simulink model "DC_motor_model"  (R2020b)
settings: Solver=ode45  StartTime=0.0  StopTime=5  RelTol=1e-3
values from neighbouring files (symbols this model uses):
  ctrl =     [DATA.mat]
  daq =     [DATA.mat]
  drv =     [DATA.mat]
  gbox =     [DATA.mat]
  mld =     [DATA.mat]
  mot =     [DATA.mat]
  rads2rpm = 9.54929658551    [DATA.mat]
  sens =     [DATA.mat]
undefined symbols (not defined in the file or in its folder): step_size
settings Model: Creator=gioel  LastModifiedBy=gioel
settings DataIOCC: ReturnWorkspaceOutputs=off

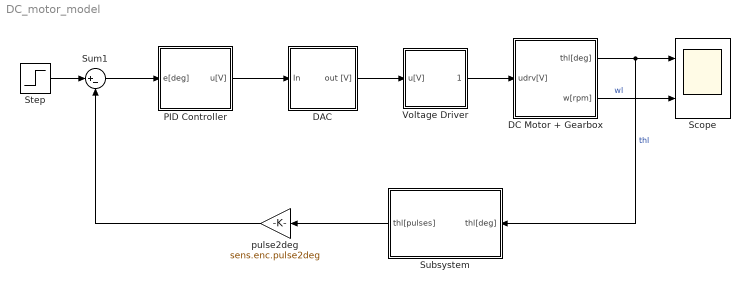
== system DC_motor_model ==
  DAC : Subsystem
  DC Motor + Gearbox : Subsystem
  PID Controller : Subsystem
  Scope : Scope  NumInputPorts=2
  Step : Step  After=step_size  SampleTime=0
  Subsystem : Subsystem
  Sum1 : Sum  Inputs=|+-
  Voltage Driver : Subsystem
  pulse2deg : Gain  Gain=sens.enc.pulse2deg
  wires:
  DAC/1(out [V]) -> Voltage Driver/1(u[V])
  Voltage Driver/1(udrv[V]) -> DC Motor + Gearbox/1(udrv[V])
  DC Motor + Gearbox/1(thl[deg]) -> Subsystem/1(thl[deg]), Scope/1  "thl"
  Subsystem/1(thl[pulses]) -> pulse2deg/1
  Sum1/1 -> PID Controller/1(e[deg])
  Step/1 -> Sum1/1
  PID Controller/1(u[V]) -> DAC/1(In)
  pulse2deg/1 -> Sum1/2
  DC Motor + Gearbox/2(w[rpm]) -> Scope/2  "wl"

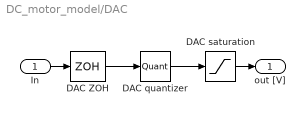
== system DC_motor_model/DAC ==
  In : Inport
  DAC quantizer : Quantizer  QuantizationInterval=daq.dac.q
  DAC saturation : Saturate  UpperLimit=daq.dac.fs  LowerLimit=-daq.dac.fs
  DAC ZOH : ZeroOrderHold  SampleTime=0.001
  out [V] : Outport
  wires:
  DAC ZOH/1 -> DAC quantizer/1
  DAC quantizer/1 -> DAC saturation/1
  In/1 -> DAC ZOH/1
  DAC saturation/1 -> out [V]/1

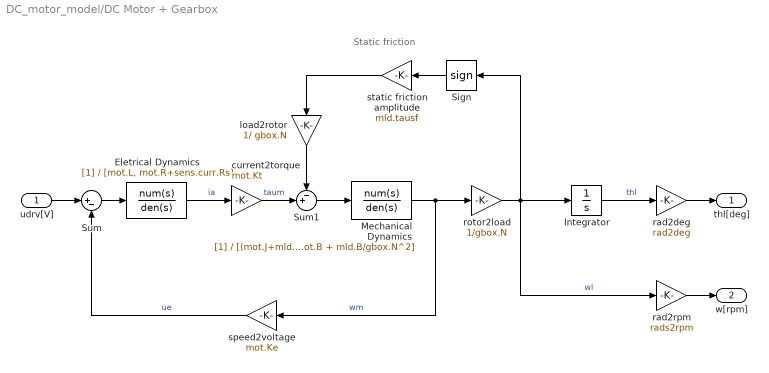
== system DC_motor_model/DC Motor + Gearbox ==
  note: Static friction
  udrv[V] : Inport
  Eletrical Dynamics : TransferFcn  Denominator=[mot.L, mot.R+sens.curr.Rs]
  Integrator : Integrator
  Mechanical Dynamics : TransferFcn  Denominator=[(mot.J+mld.J/gbox.N^2), mot.B + mld.B/gbox.N^2]
  Sign : Signum  ZeroCross=off
  Sum : Sum  Inputs=|+-
  Sum1 : Sum  Inputs=-+|
  current2torque : Gain  Gain=mot.Kt
  load2rotor : Gain  Gain=1/ gbox.N
  rad2deg : Gain  Gain=rad2deg
  "rad2rpm " : Gain  Gain=rads2rpm
  rotor2load : Gain  Gain=1/gbox.N
  speed2voltage : Gain  Gain=mot.Ke
  static friction amplitude : Gain  Gain=mld.tausf
  thl[deg] : Outport  VectorParamsAs1DForOutWhenUnconnected=off
  w[rpm] : Outport  Port=2  VectorParamsAs1DForOutWhenUnconnected=off
  wires:
  Eletrical Dynamics/1 -> current2torque/1  "ia"
  udrv[V]/1 -> Sum/1
  Sum/1 -> Eletrical Dynamics/1
  current2torque/1 -> Sum1/2  "taum"
  Sum1/1 -> Mechanical Dynamics/1
  Mechanical Dynamics/1 -> rotor2load/1, speed2voltage/1  "wm"
  rotor2load/1 -> Integrator/1, "rad2rpm "/1, Sign/1  "wl"
  Integrator/1 -> rad2deg/1  "thl"
  rad2deg/1 -> thl[deg]/1
  "rad2rpm "/1 -> w[rpm]/1
  static friction amplitude/1 -> load2rotor/1
  Sign/1 -> static friction amplitude/1
  speed2voltage/1 -> Sum/2  "ue"
  load2rotor/1 -> Sum1/1

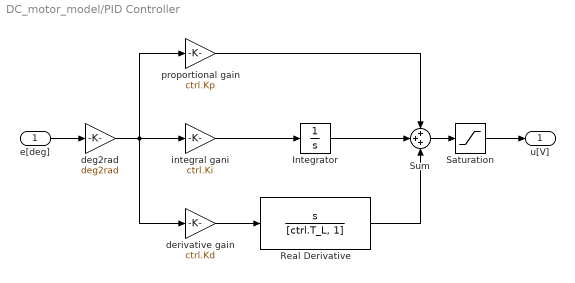
== system DC_motor_model/PID Controller ==
  e[deg] : Inport
  Integrator : Integrator
  Real Derivative : TransferFcn  Numerator=[1 0]  Denominator=[ctrl.T_L, 1]
  Saturation : Saturate  UpperLimit=drv.outmax  LowerLimit=-drv.outmax
  Sum : Sum  Inputs=+++
  deg2rad : Gain  Gain=deg2rad
  derivative gain : Gain  Gain=ctrl.Kd
  integral gani : Gain  Gain=ctrl.Ki
  proportional gain : Gain  Gain=ctrl.Kp
  u[V] : Outport
  wires:
  Sum/1 -> Saturation/1
  Saturation/1 -> u[V]/1
  derivative gain/1 -> Real Derivative/1
  Real Derivative/1 -> Sum/3
  Integrator/1 -> Sum/2
  integral gani/1 -> Integrator/1
  proportional gain/1 -> Sum/1
  e[deg]/1 -> deg2rad/1
  deg2rad/1 -> derivative gain/1, proportional gain/1, integral gani/1

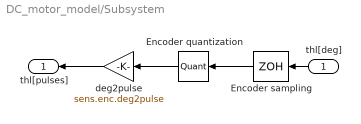
== system DC_motor_model/Subsystem ==
  thl[deg] : Inport
  Encoder quantization : Quantizer  QuantizationInterval=sens.enc.pulse2deg
  Encoder sampling : ZeroOrderHold  SampleTime=-1
  deg2pulse : Gain  Gain=sens.enc.deg2pulse
  thl[pulses] : Outport
  wires:
  thl[deg]/1 -> Encoder sampling/1
  Encoder quantization/1 -> deg2pulse/1
  Encoder sampling/1 -> Encoder quantization/1
  deg2pulse/1 -> thl[pulses]/1

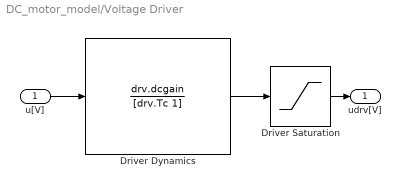
== system DC_motor_model/Voltage Driver ==
  u[V] : Inport
  Driver Dynamics : TransferFcn  Numerator=drv.dcgain  Denominator=[drv.Tc 1]
  Driver Saturation : Saturate  UpperLimit=12  LowerLimit=-12
  udrv[V] : Outport
  wires:
  Driver Dynamics/1 -> Driver Saturation/1
  Driver Saturation/1 -> udrv[V]/1
  u[V]/1 -> Driver Dynamics/1
